simulink model "SecRwRtStLgrstUpwdDnwdHolderChk"  (R2018b)
settings: Solver=FixedStepDiscrete  StartTime=0.0  StopTime=10.0  FixedStep=0.01  RelTol=1e-3
libraries: simulink x2
settings Model: Creator=sn2xws  LastModifiedBy=sn2xws
settings Model: ModifiedHistory=|
  | 2023/11/7Bug 555794 童锁需要停止 21-26
  | 25.7.7 V3.13.0 新增Md61 Md62 md30 md31
settings DataIOCC: SaveFormat=StructureWithTime
settings OptimizationCC: DefaultParameterBehavior=Inlined  EnhancedBackFolding=on  PassReuseOutputArgsAs=Individual arguments  ZeroExternalMemoryAtStartup=off  ZeroInternalMemoryAtStartup=off  OptimizeBlockOrder=speed  DifferentSizesBufferReuse=on  OptimizationCustomize=off
settings DebuggingCC: ParameterTunabilityLossMsg=error
settings ModelReferenceCC: ModelReferenceNumInstancesAllowed=Single
settings SFSimCC: MATLABDynamicMemAlloc=off
settings RTWCC: SystemTargetFile=autosar.tlc  GenCodeOnly=on  TemplateMakefile=ert_default_tmf  Description=AUTOSAR  GenerateReport=on  IncludeHyperlinkInReport=on  LaunchReport=on  GenerateTraceInfo=on  GenerateTraceReport=on  GenerateTraceReportSl=on  GenerateTraceReportSf=on  GenerateTraceReportEml=on
settings CodeAppCC: ForceParamTrailComments=on  IgnoreCustomStorageClasses=off  OperatorAnnotations=on  SimulinkDataObjDesc=on  SFDataObjDesc=on  InsertBlockDesc=on
settings STFCustomTargetCC: TargetLangStandard=C99 (ISO)  MultiwordLength=256  ParMdlRefBuildCompliant=on  CompOptLevelCompliant=on  IncludeMdlTerminateFcn=off  CombineOutputUpdateFcns=on  SuppressErrorStatus=on  ERTCustomFileBanners=on  SupportNonFinite=off  SupportComplex=off  SupportContinuousTime=off  SupportNonInlinedSFcns=off  RemoveResetFunc=on  MATLABClassNameForMDSCustomization=Simulink.SoftwareTarget.ERTCustomization  AutosarCompliant=on  UseToolchainInfoCompliant=on  LookupTableObjectStructAxisOrder=2,1,3,4,...  LUTObjectStructOrderEvenSpacing=Size,Table,Breakpoints  SystemTargetFile=autosar.tlc
settings ERTTargetCC: TargetLangStandard=C99 (ISO)  ConcurrentExecutionCompliant=off  IncludeMdlTerminateFcn=off  SuppressErrorStatus=on  SupportNonFinite=off  SupportComplex=off  ModelStepFunctionPrototypeControlCompliant=off  CPPClassGenCompliant=off  AutosarCompliant=on  LookupTableObjectStructAxisOrder=2,1,3,4,...  LUTObjectStructOrderEvenSpacing=Size,Table,Breakpoints  InlinedParameterPlacement=NonHierarchical  ERTCustomFileTemplate=example_file_process.tlc  ERTFilePackagingFormat=Compact

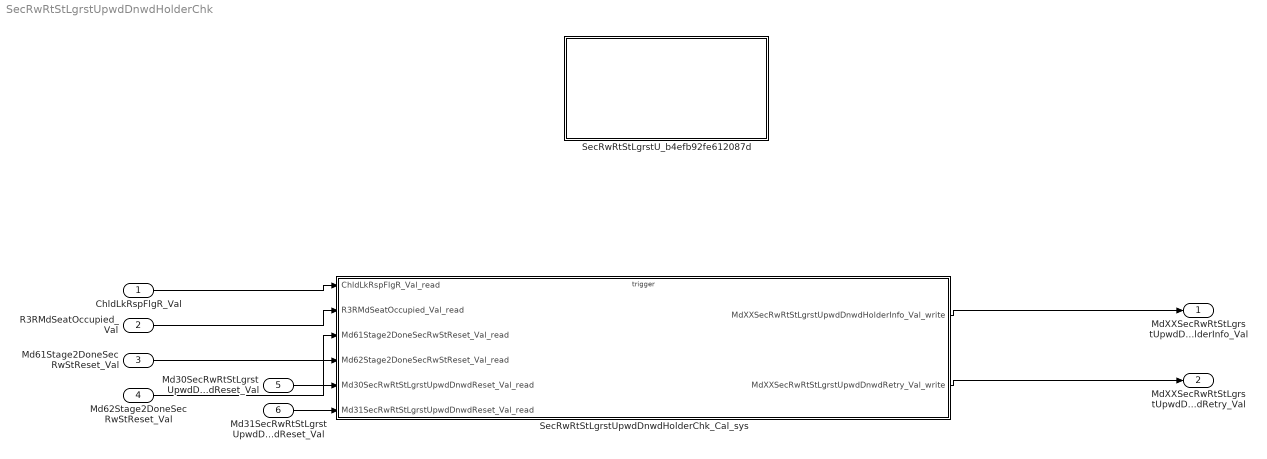
== system SecRwRtStLgrstUpwdDnwdHolderChk ==
  ChldLkRspFlgR_Val : Inport  OutDataTypeStr=boolean  PortDimensions=1
  R3RMdSeatOccupied_Val : Inport  Port=2  OutDataTypeStr=boolean  PortDimensions=1
  Md61Stage2DoneSecRwStReset_Val : Inport  Port=3  OutDataTypeStr=boolean  PortDimensions=1
  Md62Stage2DoneSecRwStReset_Val : Inport  Port=4  OutDataTypeStr=boolean  PortDimensions=1
  Md30SecRwRtStLgrstUpwdDnwdReset_Val : Inport  Port=5  OutDataTypeStr=boolean  PortDimensions=1
  Md31SecRwRtStLgrstUpwdDnwdReset_Val : Inport  Port=6  OutDataTypeStr=boolean  PortDimensions=1
  SecRwRtStLgrstU_b4efb92fe612087d : Subsystem
  SecRwRtStLgrstUpwdDnwdHolderChk_Cal_sys : Subsystem
  MdXXSecRwRtStLgrstUpwdDnwdHolderInfo_Val : Outport  OutDataTypeStr=uint32  PortDimensions=1
  MdXXSecRwRtStLgrstUpwdDnwdRetry_Val : Outport  Port=2  OutDataTypeStr=uint32  PortDimensions=1
  wires:
  ChldLkRspFlgR_Val/1 -> SecRwRtStLgrstUpwdDnwdHolderChk_Cal_sys/1(ChldLkRspFlgR_Val_read)
  R3RMdSeatOccupied_Val/1 -> SecRwRtStLgrstUpwdDnwdHolderChk_Cal_sys/2(R3RMdSeatOccupied_Val_read)
  SecRwRtStLgrstUpwdDnwdHolderChk_Cal_sys/1(MdXXSecRwRtStLgrstUpwdDnwdHolderInfo_Val_write) -> MdXXSecRwRtStLgrstUpwdDnwdHolderInfo_Val/1
  Md61Stage2DoneSecRwStReset_Val/1 -> SecRwRtStLgrstUpwdDnwdHolderChk_Cal_sys/3(Md61Stage2DoneSecRwStReset_Val_read)
  Md62Stage2DoneSecRwStReset_Val/1 -> SecRwRtStLgrstUpwdDnwdHolderChk_Cal_sys/4(Md62Stage2DoneSecRwStReset_Val_read)
  SecRwRtStLgrstUpwdDnwdHolderChk_Cal_sys/2(MdXXSecRwRtStLgrstUpwdDnwdRetry_Val_write) -> MdXXSecRwRtStLgrstUpwdDnwdRetry_Val/1
  Md30SecRwRtStLgrstUpwdDnwdReset_Val/1 -> SecRwRtStLgrstUpwdDnwdHolderChk_Cal_sys/5(Md30SecRwRtStLgrstUpwdDnwdReset_Val_read)
  Md31SecRwRtStLgrstUpwdDnwdReset_Val/1 -> SecRwRtStLgrstUpwdDnwdHolderChk_Cal_sys/6(Md31SecRwRtStLgrstUpwdDnwdReset_Val_read)

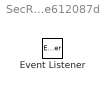
== system SecRwRtStLgrstUpwdDnwdHolderChk/SecRwRtStLgrstU_b4efb92fe612087d ==
  Event Listener : EventListener  EventName=reset

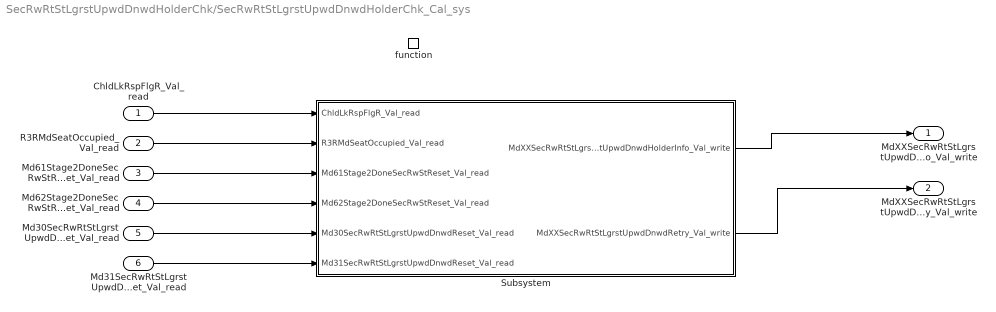
== system SecRwRtStLgrstUpwdDnwdHolderChk/SecRwRtStLgrstUpwdDnwdHolderChk_Cal_sys ==
  ChldLkRspFlgR_Val_read : Inport
  R3RMdSeatOccupied_Val_read : Inport  Port=2
  Md61Stage2DoneSecRwStReset_Val_read : Inport  Port=3
  Md62Stage2DoneSecRwStReset_Val_read : Inport  Port=4
  Md30SecRwRtStLgrstUpwdDnwdReset_Val_read : Inport  Port=5
  Md31SecRwRtStLgrstUpwdDnwdReset_Val_read : Inport  Port=6
  function : TriggerPort  TriggerType=function-call  IsSimulinkFunction=on  FunctionName=SecRwRtStLgrstUpwdDnwdHolderChk_Cal  VariantControl=(inherit)
  Subsystem : Subsystem
  MdXXSecRwRtStLgrstUpwdDnwdHolderInfo_Val_write : Outport
      settings: EnsureOutportIsVirtual=on
  MdXXSecRwRtStLgrstUpwdDnwdRetry_Val_write : Outport  Port=2
      settings: EnsureOutportIsVirtual=on
  wires:
  ChldLkRspFlgR_Val_read/1 -> Subsystem/1(ChldLkRspFlgR_Val_read)
  R3RMdSeatOccupied_Val_read/1 -> Subsystem/2(R3RMdSeatOccupied_Val_read)
  Subsystem/1(MdXXSecRwRtStLgrstUpwdDnwdHolderInfo_Val_write) -> MdXXSecRwRtStLgrstUpwdDnwdHolderInfo_Val_write/1
  Md61Stage2DoneSecRwStReset_Val_read/1 -> Subsystem/3(Md61Stage2DoneSecRwStReset_Val_read)
  Md62Stage2DoneSecRwStReset_Val_read/1 -> Subsystem/4(Md62Stage2DoneSecRwStReset_Val_read)
  Subsystem/2(MdXXSecRwRtStLgrstUpwdDnwdRetry_Val_write) -> MdXXSecRwRtStLgrstUpwdDnwdRetry_Val_write/1
  Md30SecRwRtStLgrstUpwdDnwdReset_Val_read/1 -> Subsystem/5(Md30SecRwRtStLgrstUpwdDnwdReset_Val_read)
  Md31SecRwRtStLgrstUpwdDnwdReset_Val_read/1 -> Subsystem/6(Md31SecRwRtStLgrstUpwdDnwdReset_Val_read)

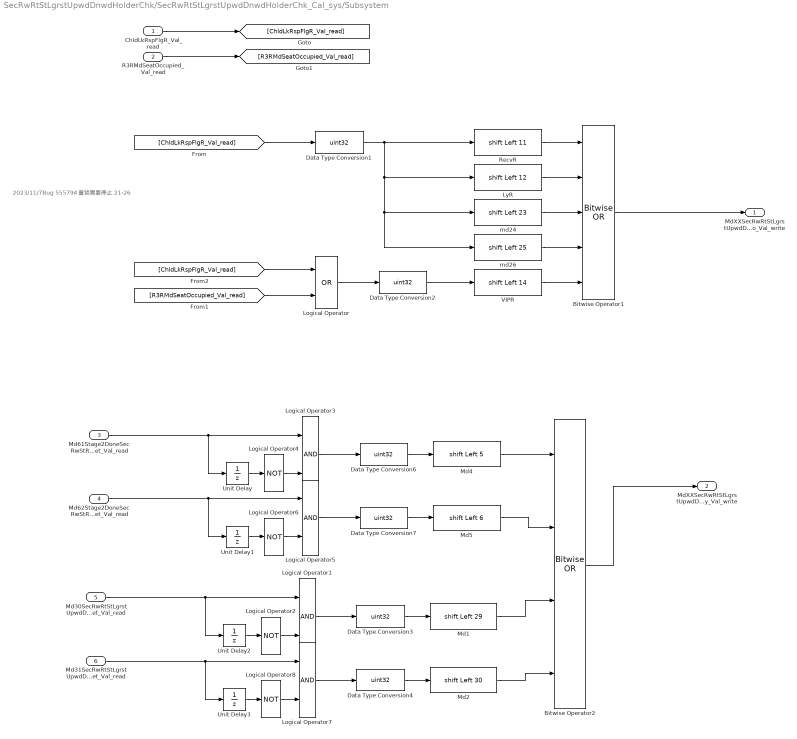
== system SecRwRtStLgrstUpwdDnwdHolderChk/SecRwRtStLgrstUpwdDnwdHolderChk_Cal_sys/Subsystem ==
  note: 2023/11/7Bug 555794 童锁需要停止 21-26
  ChldLkRspFlgR_Val_read : Inport
  R3RMdSeatOccupied_Val_read : Inport  Port=2
  Md61Stage2DoneSecRwStReset_Val_read : Inport  Port=3
  Md62Stage2DoneSecRwStReset_Val_read : Inport  Port=4
  Md30SecRwRtStLgrstUpwdDnwdReset_Val_read : Inport  Port=5
  Md31SecRwRtStLgrstUpwdDnwdReset_Val_read : Inport  Port=6
  Bitwise Operator1 : simulink/Logic and Bit Operations/Bitwise Operator  logicop=OR  UseBitMask=off  NumInputPorts=5  BitMask=bin2dec('11011001')  BitMaskRealWorld=Stored Integer
  Bitwise Operator2 : simulink/Logic and Bit Operations/Bitwise Operator  logicop=OR  UseBitMask=off  NumInputPorts=4  BitMask=bin2dec('11011001')  BitMaskRealWorld=Stored Integer
  Data Type Conversion{1..4,6..7} (6 alike) : DataTypeConversion  OutDataTypeStr=uint32
  Logical Operator : Logic  Operator=OR  AllPortsSameDT=off  OutDataTypeStr=boolean
  Logical Operator{1,3,5,7} (4 alike) : Logic  AllPortsSameDT=off  OutDataTypeStr=boolean
  Logical Operator{2,4,6,8} (4 alike) : Logic  Operator=NOT  AllPortsSameDT=off  OutDataTypeStr=boolean
  LyR : ArithShift  BitShiftNumber=12  BitShiftDirection=Left
  Md1 : ArithShift  BitShiftNumber=29  BitShiftDirection=Left
  Md2 : ArithShift  BitShiftNumber=30  BitShiftDirection=Left
  Md4 : ArithShift  BitShiftNumber=5  BitShiftDirection=Left
  Md5 : ArithShift  BitShiftNumber=6  BitShiftDirection=Left
  RecvR : ArithShift  BitShiftNumber=11  BitShiftDirection=Left
  Unit Delay{,1..3} (4 alike) : UnitDelay  SampleTime=-1
  VIPR : ArithShift  BitShiftNumber=14  BitShiftDirection=Left
  md24 : ArithShift  BitShiftNumber=23  BitShiftDirection=Left
  md26 : ArithShift  BitShiftNumber=25  BitShiftDirection=Left
  MdXXSecRwRtStLgrstUpwdDnwdHolderInfo_Val_write : Outport
      settings: EnsureOutportIsVirtual=on
  MdXXSecRwRtStLgrstUpwdDnwdRetry_Val_write : Outport  Port=2
      settings: EnsureOutportIsVirtual=on
  wires:
  ChldLkRspFlgR_Val_read/1 -> [ChldLkRspFlgR_Val_read]
  R3RMdSeatOccupied_Val_read/1 -> [R3RMdSeatOccupied_Val_read]
  Bitwise Operator1/1 -> MdXXSecRwRtStLgrstUpwdDnwdHolderInfo_Val_write/1
  Data Type Conversion1/1 -> RecvR/1, md26/1, md24/1, LyR/1
  RecvR/1 -> Bitwise Operator1/1
  LyR/1 -> Bitwise Operator1/2
  [ChldLkRspFlgR_Val_read] -> Data Type Conversion1/1
  [ChldLkRspFlgR_Val_read] -> Logical Operator/1
  [R3RMdSeatOccupied_Val_read] -> Logical Operator/2
  Data Type Conversion2/1 -> VIPR/1
  Logical Operator/1 -> Data Type Conversion2/1
  VIPR/1 -> Bitwise Operator1/5
  md24/1 -> Bitwise Operator1/3
  md26/1 -> Bitwise Operator1/4
  Data Type Conversion7/1 -> Md5/1
  Logical Operator5/1 -> Data Type Conversion7/1
  Logical Operator6/1 -> Logical Operator5/2
  Unit Delay/1 -> Logical Operator4/1
  Md5/1 -> Bitwise Operator2/2
  Data Type Conversion6/1 -> Md4/1
  Md4/1 -> Bitwise Operator2/1
  Logical Operator3/1 -> Data Type Conversion6/1
  Logical Operator4/1 -> Logical Operator3/2
  Unit Delay1/1 -> Logical Operator6/1
  Md62Stage2DoneSecRwStReset_Val_read/1 -> Logical Operator5/1, Unit Delay1/1
  Bitwise Operator2/1 -> MdXXSecRwRtStLgrstUpwdDnwdRetry_Val_write/1
  Md61Stage2DoneSecRwStReset_Val_read/1 -> Logical Operator3/1, Unit Delay/1
  Md30SecRwRtStLgrstUpwdDnwdReset_Val_read/1 -> Unit Delay2/1, Logical Operator1/1
  Md31SecRwRtStLgrstUpwdDnwdReset_Val_read/1 -> Unit Delay3/1, Logical Operator7/1
  Unit Delay3/1 -> Logical Operator8/1
  Logical Operator2/1 -> Logical Operator1/2
  Logical Operator1/1 -> Data Type Conversion3/1
  Md1/1 -> Bitwise Operator2/3
  Data Type Conversion3/1 -> Md1/1
  Md2/1 -> Bitwise Operator2/4
  Unit Delay2/1 -> Logical Operator2/1
  Logical Operator8/1 -> Logical Operator7/2
  Logical Operator7/1 -> Data Type Conversion4/1
  Data Type Conversion4/1 -> Md2/1
